simulink model "random_number_spectrum"  (R2024a)
settings: Solver=VariableStepAuto  StartTime=0.0  StopTime=50.0  RelTol=1e-3
libraries: simulink_extras x4
settings Model: Creator=evgenijkondratev  LastModifiedBy=evgenijkondratev

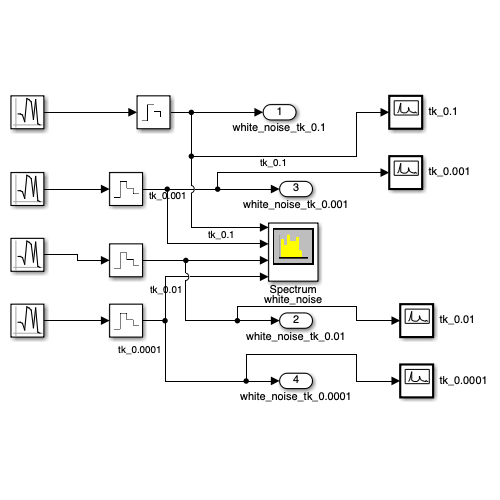
[thumbnail: Simulink's stored preview of the top-level diagram]
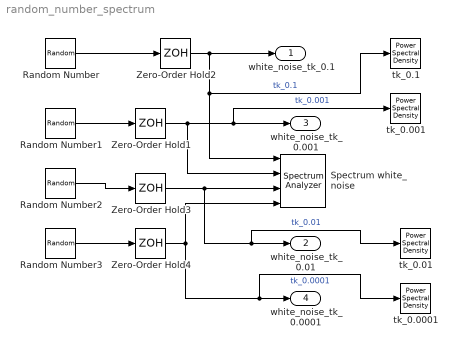
== system random_number_spectrum ==
  Random Number : RandomNumber  SampleTime=0.1
  Random Number1 : RandomNumber  SampleTime=0.001
  Random Number2 : RandomNumber  SampleTime=0.01
  Random Number3 : RandomNumber  SampleTime=0.0001
  Spectrum white_noise : SpectrumAnalyzer  NumInputPorts=4  WindowPosition=[170.000000,173.000000,1565.000000,787.000000,]  ScopeFrameLocation=window  YLimits=[-60.99615924,28.34718874]  ShowLegend=on
  Zero-Order Hold{1..4} (4 alike) : ZeroOrderHold  SampleTime=0.001
  tk_0.0001 : simulink_extras/Additional Sinks/Power Spectral Density  npts=128  fftpts=512  HowOften=64  sampleT=0.1
  tk_0.001 : simulink_extras/Additional Sinks/Power Spectral Density  npts=128  fftpts=512  HowOften=64  sampleT=0.1
  tk_0.01 : simulink_extras/Additional Sinks/Power Spectral Density  npts=128  fftpts=512  HowOften=64  sampleT=0.1
  tk_0.1 : simulink_extras/Additional Sinks/Power Spectral Density  npts=128  fftpts=512  HowOften=64  sampleT=0.1
  white_noise_tk_0.1 : Outport
  white_noise_tk_0.01 : Outport  Port=2
  white_noise_tk_0.001 : Outport  Port=3
  white_noise_tk_0.0001 : Outport  Port=4
  wires:
  Zero-Order Hold1/1 -> tk_0.001/1, white_noise_tk_0.001/1, Spectrum white_noise/2  "tk_0.001"
  Zero-Order Hold2/1 -> tk_0.1/1, Spectrum white_noise/1, white_noise_tk_0.1/1  "tk_0.1"
  Zero-Order Hold3/1 -> tk_0.01/1, white_noise_tk_0.01/1, Spectrum white_noise/3  "tk_0.01"
  Random Number/1 -> Zero-Order Hold2/1
  Random Number2/1 -> Zero-Order Hold3/1
  Random Number3/1 -> Zero-Order Hold4/1
  Random Number1/1 -> Zero-Order Hold1/1
  Zero-Order Hold4/1 -> tk_0.0001/1, white_noise_tk_0.0001/1, Spectrum white_noise/4  "tk_0.0001"
